simulink model "ForceCoordinateTransform"  (R2026b)
settings: Solver=ode45  StopTime=1
settings Model: Creator=Xu Dingyi  LastModifiedBy=29358

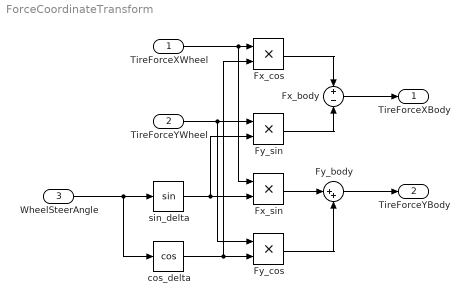
== system ForceCoordinateTransform ==
  TireForceXWheel : Inport  OutDataTypeStr=double  PortDimensions=[4 1]
  TireForceYWheel : Inport  Port=2  OutDataTypeStr=double  PortDimensions=[4 1]
  WheelSteerAngle : Inport  Port=3  OutDataTypeStr=double  PortDimensions=[4 1]
  Fx_body : Sum  Inputs=+-
  Fx_cos : Product  Inputs=**
  Fx_sin : Product  Inputs=**
  Fy_body : Sum  Inputs=|++
  Fy_cos : Product  Inputs=**
  Fy_sin : Product  Inputs=**
  cos_delta : Trigonometry  Operator=cos
  sin_delta : Trigonometry
  TireForceXBody : Outport
  TireForceYBody : Outport  Port=2
  wires:
  WheelSteerAngle/1 -> cos_delta/1, sin_delta/1
  TireForceXWheel/1 -> Fx_cos/1, Fx_sin/1
  TireForceYWheel/1 -> Fy_sin/1, Fy_cos/1
  sin_delta/1 -> Fy_sin/2, Fx_sin/2
  cos_delta/1 -> Fx_cos/2, Fy_cos/2
  Fx_sin/1 -> Fy_body/1
  Fx_cos/1 -> Fx_body/1
  Fy_sin/1 -> Fx_body/2
  Fy_cos/1 -> Fy_body/2
  Fx_body/1 -> TireForceXBody/1
  Fy_body/1 -> TireForceYBody/1
